simulink model "Drone_Model"  (R2021a)
settings: Solver=VariableStepAuto  StartTime=0.0  StopTime=10.0  MaxStep=1e-4  RelTol=1e-3
values from neighbouring files (symbols this model uses):
  g = 9.81    [Parameters.m]
  m = 0.8    [Parameters.m]
  Omega_sq_2_U = [b  b  b  b ... (first row only)    [Parameters.m]
  p1 = (Iyy-Izz)/Ixx    (= -0.808551372049)    [Parameters.m]
  p3 = l/Ixx    (= 19.1448627951)    [Parameters.m]
  p4 = (Izz-Ixx)/Iyy    (= 0.808551372049)    [Parameters.m]
  p6 = l/Iyy    (= 19.1448627951)    [Parameters.m]
  p7 = (Ixx-Iyy)/Izz    (= 0)    [Parameters.m]
  phi_0 = 0    [Parameters.m]
  phi_dot_0 = 0    [Parameters.m]
  psi_0 = 0    [Parameters.m]
  psi_dot_0 = 0    [Parameters.m]
  th_0 = 0    [Parameters.m]
  th_dot_0 = 0    [Parameters.m]
  U_Sq_max = U_max^2    (= 2467401.10027)    [Parameters.m]
  U_to_Omega_sq = inv(Omega_sq_2_U)    [Parameters.m]
  x_0 = 0.1    [Parameters.m]
  x_dot_0 = 0    [Parameters.m]
  y_0 = 0    [Parameters.m]
  y_dot_0 = 0    [Parameters.m]
  z_0 = 0    [Parameters.m]
  z_dot_0 = 0    [Parameters.m]
libraries: pid_lib x5
settings Model: Creator=jkord  LastModifiedBy=nikol
settings DebuggingCC: UnconnectedInputMsg=none  UnconnectedOutputMsg=none  UnconnectedLineMsg=none
settings ModelReferenceCC: EnableRefExpFcnMdlSchedulingChecks=off
settings RTWCC: Description=Generic Real-Time Target  GPUComputeCapability=5.0  DLArmComputeVersion=20.02.1

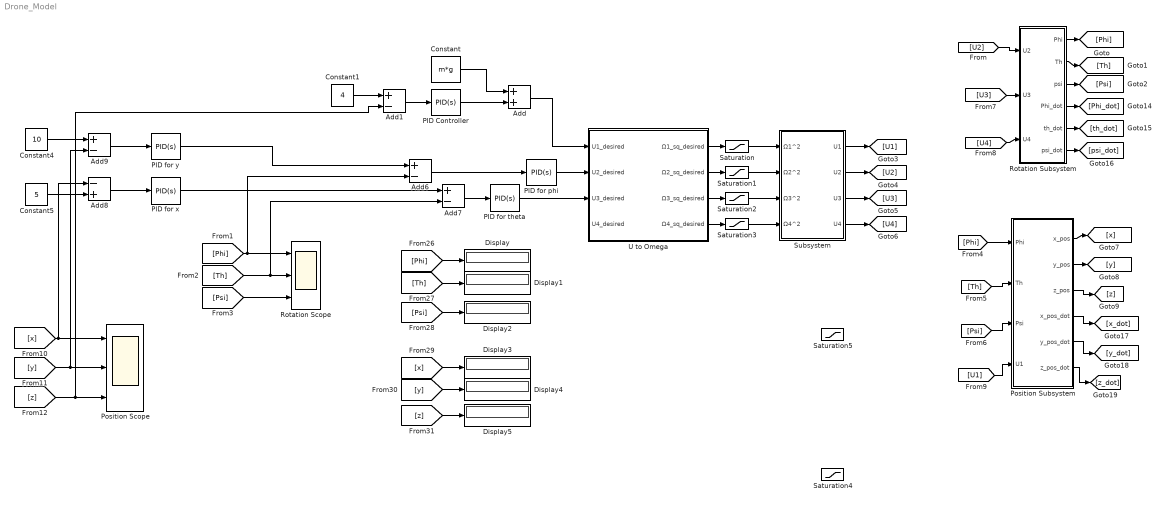
== system Drone_Model ==
  Add : Sum
  Add{1,6..7,9} (4 alike) : Sum  Inputs=+-
  Add8 : Sum  Inputs=-+
  Constant : Constant  Value=m*g
  Constant1 : Constant  Value=4
  Constant4 : Constant  Value=10
  Constant5 : Constant  Value=5
  Display{,1..5} (6 alike) : Display
  PID Controller : pid_lib/PID Controller  Controller=PID  Form=Parallel  TimeDomain=Continuous-time  UseExternalTs=off  SampleTime=-1  IntegratorMethod=Forward Euler  FilterMethod=Forward Euler  ControllerParametersSource=internal  P=0.81  I=0.875  D=0.9  UseFilter=on  N=100  TunerSelectOption=Frequency Response Based  InitialConditionSource=internal  InitialConditionForIntegrator=0  InitialConditionForFilter=0  DifferentiatorICPrevScaledInput=0  ExternalReset=none  TrackingMode=off  Kt=1  LimitOutput=off  SatLimitsSource=internal  UpperSaturationLimit=inf  LowerSaturationLimit=-inf  LinearizeAsGain=on  AntiWindupMode=none  Kb=1  POutMin=[]  POutMax=[]  IOutMin=[]  IOutMax=[]  DOutMin=[]  DOutMax=[]  NOutMin=[]  NOutMax=[]  SumOutMin=[]  SumOutMax=[]  SaturationOutMin=[]  SaturationOutMax=[]  PParamMin=[]  PParamMax=[]  IParamMin=[]  IParamMax=[]  DParamMin=[]  DParamMax=[]  NParamMin=[]  NParamMax=[]  KbParamMin=[]  KbParamMax=[]  KtParamMin=[]  KtParamMax=[]  KbOutMin=[]  KbOutMax=[]  KtOutMin=[]  KtOutMax=[]  IntegratorOutMin=[]  IntegratorOutMax=[]  FilterOutMin=[]  FilterOutMax=[]  SumI1OutMin=[]  SumI1OutMax=[]  SumI2OutMin=[]  SumI2OutMax=[]  SumI3OutMin=[]  SumI3OutMax=[]  SumI4OutMin=[]  SumI4OutMax=[]  SumDOutMin=[]  SumDOutMax=[]  DifferentiatorOutMin=[]  DifferentiatorOutMax=[]  FilterDiffOutCoefMin=[]  FilterDiffOutCoefMax=[]  ReciprocalOutMin=[]  ReciprocalOutMax=[]  SumDenOutMin=[]  SumDenOutMax=[]  SumNumOutMin=[]  SumNumOutMax=[]  DivideOutMin=[]  DivideOutMax=[]  UdiffTsProdOutMin=[]  UdiffTsProdOutMax=[]  NTsProdOutMin=[]  NTsProdOutMax=[]  UintegralTsProdOutMin=[]  UintegralTsProdOutMax=[]  UngainTsProdOutMin=[]  UngainTsProdOutMax=[]  IntegratorContinuousStateAttributes=''  IntegratorStateMustResolveToSignalObject=off  IntegratorRTWStateStorageClass=Auto  FilterContinuousStateAttributes=''  FilterStateMustResolveToSignalObject=off  FilterRTWStateStorageClass=Auto  ParallelPVariant=InternalParameters  IdealPVariant=Disabled  IVariant=InternalParameters  DVariant=InternalParameters  IntegratorVariant=Continuous  SatVariant=Disabled  AWVariant=Passthrough  PCopyVariant=Disabled  TRVariant=Disabled  FdbkBlocksVariant=Forward  IdealPFdbkVariant=Disabled  SatFdbkVariant=Disabled  DerivativeFilterVariant=ContFilter  NVariant=InternalParameters  NCopyVariant=Disabled  FilterICVariant=InternalICsFilter  IntegratorICVariant=InternalICs  ExternalResetVariant=Disabled  TRSumVariant=Passthrough  SumFdbkVariant=Disabled  SumVariant=Sum_PID  TsampFilterVariant=InternalTs  TsampNgainVariant=Passthrough  TsampIntegralVariant=Passthrough  ExternalSaturationOutDataTypeStr=Inherit: Same as second input
  PID for phi : pid_lib/PID Controller  Controller=PID  Form=Parallel  TimeDomain=Continuous-time  UseExternalTs=off  SampleTime=-1  IntegratorMethod=Forward Euler  FilterMethod=Forward Euler  ControllerParametersSource=internal  P=1  I=0.01  D=0.5  UseFilter=on  N=100  TunerSelectOption=Frequency Response Based  InitialConditionSource=internal  InitialConditionForIntegrator=0  InitialConditionForFilter=0  DifferentiatorICPrevScaledInput=0  ExternalReset=none  TrackingMode=off  Kt=1  LimitOutput=off  SatLimitsSource=internal  UpperSaturationLimit=inf  LowerSaturationLimit=-inf  LinearizeAsGain=on  AntiWindupMode=none  Kb=1  POutMin=[]  POutMax=[]  IOutMin=[]  IOutMax=[]  DOutMin=[]  DOutMax=[]  NOutMin=[]  NOutMax=[]  SumOutMin=[]  SumOutMax=[]  SaturationOutMin=[]  SaturationOutMax=[]  PParamMin=[]  PParamMax=[]  IParamMin=[]  IParamMax=[]  DParamMin=[]  DParamMax=[]  NParamMin=[]  NParamMax=[]  KbParamMin=[]  KbParamMax=[]  KtParamMin=[]  KtParamMax=[]  KbOutMin=[]  KbOutMax=[]  KtOutMin=[]  KtOutMax=[]  IntegratorOutMin=[]  IntegratorOutMax=[]  FilterOutMin=[]  FilterOutMax=[]  SumI1OutMin=[]  SumI1OutMax=[]  SumI2OutMin=[]  SumI2OutMax=[]  SumI3OutMin=[]  SumI3OutMax=[]  SumI4OutMin=[]  SumI4OutMax=[]  SumDOutMin=[]  SumDOutMax=[]  DifferentiatorOutMin=[]  DifferentiatorOutMax=[]  FilterDiffOutCoefMin=[]  FilterDiffOutCoefMax=[]  ReciprocalOutMin=[]  ReciprocalOutMax=[]  SumDenOutMin=[]  SumDenOutMax=[]  SumNumOutMin=[]  SumNumOutMax=[]  DivideOutMin=[]  DivideOutMax=[]  UdiffTsProdOutMin=[]  UdiffTsProdOutMax=[]  NTsProdOutMin=[]  NTsProdOutMax=[]  UintegralTsProdOutMin=[]  UintegralTsProdOutMax=[]  UngainTsProdOutMin=[]  UngainTsProdOutMax=[]  IntegratorContinuousStateAttributes=''  IntegratorStateMustResolveToSignalObject=off  IntegratorRTWStateStorageClass=Auto  FilterContinuousStateAttributes=''  FilterStateMustResolveToSignalObject=off  FilterRTWStateStorageClass=Auto  ParallelPVariant=InternalParameters  IdealPVariant=Disabled  IVariant=InternalParameters  DVariant=InternalParameters  IntegratorVariant=Continuous  SatVariant=Disabled  AWVariant=Passthrough  PCopyVariant=Disabled  TRVariant=Disabled  FdbkBlocksVariant=Forward  IdealPFdbkVariant=Disabled  SatFdbkVariant=Disabled  DerivativeFilterVariant=ContFilter  NVariant=InternalParameters  NCopyVariant=Disabled  FilterICVariant=InternalICsFilter  IntegratorICVariant=InternalICs  ExternalResetVariant=Disabled  TRSumVariant=Passthrough  SumFdbkVariant=Disabled  SumVariant=Sum_PID  TsampFilterVariant=InternalTs  TsampNgainVariant=Passthrough  TsampIntegralVariant=Passthrough  ExternalSaturationOutDataTypeStr=Inherit: Same as second input
  PID for theta : pid_lib/PID Controller  Controller=PID  Form=Parallel  TimeDomain=Continuous-time  UseExternalTs=off  SampleTime=-1  IntegratorMethod=Forward Euler  FilterMethod=Forward Euler  ControllerParametersSource=internal  P=0.75  I=0.16  D=0.12  UseFilter=on  N=100  TunerSelectOption=Frequency Response Based  InitialConditionSource=internal  InitialConditionForIntegrator=0  InitialConditionForFilter=0  DifferentiatorICPrevScaledInput=0  ExternalReset=none  TrackingMode=off  Kt=1  LimitOutput=off  SatLimitsSource=internal  UpperSaturationLimit=inf  LowerSaturationLimit=-inf  LinearizeAsGain=on  AntiWindupMode=none  Kb=1  POutMin=[]  POutMax=[]  IOutMin=[]  IOutMax=[]  DOutMin=[]  DOutMax=[]  NOutMin=[]  NOutMax=[]  SumOutMin=[]  SumOutMax=[]  SaturationOutMin=[]  SaturationOutMax=[]  PParamMin=[]  PParamMax=[]  IParamMin=[]  IParamMax=[]  DParamMin=[]  DParamMax=[]  NParamMin=[]  NParamMax=[]  KbParamMin=[]  KbParamMax=[]  KtParamMin=[]  KtParamMax=[]  KbOutMin=[]  KbOutMax=[]  KtOutMin=[]  KtOutMax=[]  IntegratorOutMin=[]  IntegratorOutMax=[]  FilterOutMin=[]  FilterOutMax=[]  SumI1OutMin=[]  SumI1OutMax=[]  SumI2OutMin=[]  SumI2OutMax=[]  SumI3OutMin=[]  SumI3OutMax=[]  SumI4OutMin=[]  SumI4OutMax=[]  SumDOutMin=[]  SumDOutMax=[]  DifferentiatorOutMin=[]  DifferentiatorOutMax=[]  FilterDiffOutCoefMin=[]  FilterDiffOutCoefMax=[]  ReciprocalOutMin=[]  ReciprocalOutMax=[]  SumDenOutMin=[]  SumDenOutMax=[]  SumNumOutMin=[]  SumNumOutMax=[]  DivideOutMin=[]  DivideOutMax=[]  UdiffTsProdOutMin=[]  UdiffTsProdOutMax=[]  NTsProdOutMin=[]  NTsProdOutMax=[]  UintegralTsProdOutMin=[]  UintegralTsProdOutMax=[]  UngainTsProdOutMin=[]  UngainTsProdOutMax=[]  IntegratorContinuousStateAttributes=''  IntegratorStateMustResolveToSignalObject=off  IntegratorRTWStateStorageClass=Auto  FilterContinuousStateAttributes=''  FilterStateMustResolveToSignalObject=off  FilterRTWStateStorageClass=Auto  ParallelPVariant=InternalParameters  IdealPVariant=Disabled  IVariant=InternalParameters  DVariant=InternalParameters  IntegratorVariant=Continuous  SatVariant=Disabled  AWVariant=Passthrough  PCopyVariant=Disabled  TRVariant=Disabled  FdbkBlocksVariant=Forward  IdealPFdbkVariant=Disabled  SatFdbkVariant=Disabled  DerivativeFilterVariant=ContFilter  NVariant=InternalParameters  NCopyVariant=Disabled  FilterICVariant=InternalICsFilter  IntegratorICVariant=InternalICs  ExternalResetVariant=Disabled  TRSumVariant=Passthrough  SumFdbkVariant=Disabled  SumVariant=Sum_PID  TsampFilterVariant=InternalTs  TsampNgainVariant=Passthrough  TsampIntegralVariant=Passthrough  ExternalSaturationOutDataTypeStr=Inherit: Same as second input
  PID for x : pid_lib/PID Controller  Controller=PID  Form=Parallel  TimeDomain=Continuous-time  UseExternalTs=off  SampleTime=-1  IntegratorMethod=Forward Euler  FilterMethod=Forward Euler  ControllerParametersSource=internal  P=1  I=.01  D=.25  UseFilter=on  N=100  TunerSelectOption=Frequency Response Based  InitialConditionSource=internal  InitialConditionForIntegrator=0  InitialConditionForFilter=0  DifferentiatorICPrevScaledInput=0  ExternalReset=none  TrackingMode=off  Kt=1  LimitOutput=off  SatLimitsSource=internal  UpperSaturationLimit=inf  LowerSaturationLimit=-inf  LinearizeAsGain=on  AntiWindupMode=none  Kb=1  POutMin=[]  POutMax=[]  IOutMin=[]  IOutMax=[]  DOutMin=[]  DOutMax=[]  NOutMin=[]  NOutMax=[]  SumOutMin=[]  SumOutMax=[]  SaturationOutMin=[]  SaturationOutMax=[]  PParamMin=[]  PParamMax=[]  IParamMin=[]  IParamMax=[]  DParamMin=[]  DParamMax=[]  NParamMin=[]  NParamMax=[]  KbParamMin=[]  KbParamMax=[]  KtParamMin=[]  KtParamMax=[]  KbOutMin=[]  KbOutMax=[]  KtOutMin=[]  KtOutMax=[]  IntegratorOutMin=[]  IntegratorOutMax=[]  FilterOutMin=[]  FilterOutMax=[]  SumI1OutMin=[]  SumI1OutMax=[]  SumI2OutMin=[]  SumI2OutMax=[]  SumI3OutMin=[]  SumI3OutMax=[]  SumI4OutMin=[]  SumI4OutMax=[]  SumDOutMin=[]  SumDOutMax=[]  DifferentiatorOutMin=[]  DifferentiatorOutMax=[]  FilterDiffOutCoefMin=[]  FilterDiffOutCoefMax=[]  ReciprocalOutMin=[]  ReciprocalOutMax=[]  SumDenOutMin=[]  SumDenOutMax=[]  SumNumOutMin=[]  SumNumOutMax=[]  DivideOutMin=[]  DivideOutMax=[]  UdiffTsProdOutMin=[]  UdiffTsProdOutMax=[]  NTsProdOutMin=[]  NTsProdOutMax=[]  UintegralTsProdOutMin=[]  UintegralTsProdOutMax=[]  UngainTsProdOutMin=[]  UngainTsProdOutMax=[]  IntegratorContinuousStateAttributes=''  IntegratorStateMustResolveToSignalObject=off  IntegratorRTWStateStorageClass=Auto  FilterContinuousStateAttributes=''  FilterStateMustResolveToSignalObject=off  FilterRTWStateStorageClass=Auto  ParallelPVariant=InternalParameters  IdealPVariant=Disabled  IVariant=InternalParameters  DVariant=InternalParameters  IntegratorVariant=Continuous  SatVariant=Disabled  AWVariant=Passthrough  PCopyVariant=Disabled  TRVariant=Disabled  FdbkBlocksVariant=Forward  IdealPFdbkVariant=Disabled  SatFdbkVariant=Disabled  DerivativeFilterVariant=ContFilter  NVariant=InternalParameters  NCopyVariant=Disabled  FilterICVariant=InternalICsFilter  IntegratorICVariant=InternalICs  ExternalResetVariant=Disabled  TRSumVariant=Passthrough  SumFdbkVariant=Disabled  SumVariant=Sum_PID  TsampFilterVariant=InternalTs  TsampNgainVariant=Passthrough  TsampIntegralVariant=Passthrough  ExternalSaturationOutDataTypeStr=Inherit: Same as second input
  PID for y : pid_lib/PID Controller  Controller=PID  Form=Parallel  TimeDomain=Continuous-time  UseExternalTs=off  SampleTime=-1  IntegratorMethod=Forward Euler  FilterMethod=Forward Euler  ControllerParametersSource=internal  P=0.6  I=0  D=0.3  UseFilter=on  N=100  TunerSelectOption=Frequency Response Based  InitialConditionSource=internal  InitialConditionForIntegrator=0  InitialConditionForFilter=0  DifferentiatorICPrevScaledInput=0  ExternalReset=none  TrackingMode=off  Kt=1  LimitOutput=off  SatLimitsSource=internal  UpperSaturationLimit=inf  LowerSaturationLimit=-inf  LinearizeAsGain=on  AntiWindupMode=none  Kb=1  POutMin=[]  POutMax=[]  IOutMin=[]  IOutMax=[]  DOutMin=[]  DOutMax=[]  NOutMin=[]  NOutMax=[]  SumOutMin=[]  SumOutMax=[]  SaturationOutMin=[]  SaturationOutMax=[]  PParamMin=[]  PParamMax=[]  IParamMin=[]  IParamMax=[]  DParamMin=[]  DParamMax=[]  NParamMin=[]  NParamMax=[]  KbParamMin=[]  KbParamMax=[]  KtParamMin=[]  KtParamMax=[]  KbOutMin=[]  KbOutMax=[]  KtOutMin=[]  KtOutMax=[]  IntegratorOutMin=[]  IntegratorOutMax=[]  FilterOutMin=[]  FilterOutMax=[]  SumI1OutMin=[]  SumI1OutMax=[]  SumI2OutMin=[]  SumI2OutMax=[]  SumI3OutMin=[]  SumI3OutMax=[]  SumI4OutMin=[]  SumI4OutMax=[]  SumDOutMin=[]  SumDOutMax=[]  DifferentiatorOutMin=[]  DifferentiatorOutMax=[]  FilterDiffOutCoefMin=[]  FilterDiffOutCoefMax=[]  ReciprocalOutMin=[]  ReciprocalOutMax=[]  SumDenOutMin=[]  SumDenOutMax=[]  SumNumOutMin=[]  SumNumOutMax=[]  DivideOutMin=[]  DivideOutMax=[]  UdiffTsProdOutMin=[]  UdiffTsProdOutMax=[]  NTsProdOutMin=[]  NTsProdOutMax=[]  UintegralTsProdOutMin=[]  UintegralTsProdOutMax=[]  UngainTsProdOutMin=[]  UngainTsProdOutMax=[]  IntegratorContinuousStateAttributes=''  IntegratorStateMustResolveToSignalObject=off  IntegratorRTWStateStorageClass=Auto  FilterContinuousStateAttributes=''  FilterStateMustResolveToSignalObject=off  FilterRTWStateStorageClass=Auto  ParallelPVariant=InternalParameters  IdealPVariant=Disabled  IVariant=InternalParameters  DVariant=InternalParameters  IntegratorVariant=Continuous  SatVariant=Disabled  AWVariant=Passthrough  PCopyVariant=Disabled  TRVariant=Disabled  FdbkBlocksVariant=Forward  IdealPFdbkVariant=Disabled  SatFdbkVariant=Disabled  DerivativeFilterVariant=ContFilter  NVariant=InternalParameters  NCopyVariant=Disabled  FilterICVariant=InternalICsFilter  IntegratorICVariant=InternalICs  ExternalResetVariant=Disabled  TRSumVariant=Passthrough  SumFdbkVariant=Disabled  SumVariant=Sum_PID  TsampFilterVariant=InternalTs  TsampNgainVariant=Passthrough  TsampIntegralVariant=Passthrough  ExternalSaturationOutDataTypeStr=Inherit: Same as second input
  Position Subsystem : Subsystem
  Position Scope : Scope  NumInputPorts=3
  Rotation Subsystem : Subsystem
  Rotation Scope : Scope  NumInputPorts=3
  Saturation{,1..5} (6 alike) : Saturate  UpperLimit=U_Sq_max  LowerLimit=0
  Subsystem : Subsystem
  U to Omega : Subsystem
  wires:
  [Th] -> Position Subsystem/2(Th)
  [U3] -> Rotation Subsystem/2(U3)
  Rotation Subsystem/3(psi) -> [Psi]
  [U4] -> Rotation Subsystem/3(U4)
  Rotation Subsystem/1(Phi) -> [Phi]
  Rotation Subsystem/6(psi_dot) -> [psi_dot]
  Rotation Subsystem/2(Th) -> [Th]
  Position Subsystem/6(z_pos_dot) -> [z_dot]
  [Phi] -> Position Subsystem/1(Phi)
  Rotation Subsystem/4(Phi_dot) -> [Phi_dot]
  Rotation Subsystem/5(th_dot) -> [th_dot]
  Position Subsystem/4(x_pos_dot) -> [x_dot]
  [Psi] -> Position Subsystem/3(Psi)
  Position Subsystem/5(y_pos_dot) -> [y_dot]
  Position Subsystem/1(x_pos) -> [x]
  [U1] -> Position Subsystem/4(U1)
  Position Subsystem/3(z_pos) -> [z]
  Position Subsystem/2(y_pos) -> [y]
  [U2] -> Rotation Subsystem/1(U2)
  U to Omega/1(Ω1_sq_desired) -> Saturation/1
  Saturation3/1 -> Subsystem/4(Ω4^2)
  U to Omega/3(Ω3_sq_desired) -> Saturation2/1
  U to Omega/2(Ω2_sq_desired) -> Saturation1/1
  Saturation2/1 -> Subsystem/3(Ω3^2)
  Saturation1/1 -> Subsystem/2(Ω2^2)
  U to Omega/4(Ω4_sq_desired) -> Saturation3/1
  Subsystem/4(U4) -> [U4]
  Saturation/1 -> Subsystem/1(Ω1^2)
  Subsystem/2(U2) -> [U2]
  Subsystem/3(U3) -> [U3]
  Subsystem/1(U1) -> [U1]
  [Psi] -> Rotation Scope/3
  [z] -> Display5/1
  [Psi] -> Display2/1
  [Th] -> Display1/1
  [Phi] -> Display/1
  [x] -> Display3/1
  [y] -> Display4/1
  PID Controller/1 -> Add/2
  Constant/1 -> Add/1
  Add1/1 -> PID Controller/1
  Constant1/1 -> Add1/1
  [z] -> Add1/2, Position Scope/3
  Add/1 -> U to Omega/1(U1_desired)
  PID for theta/1 -> U to Omega/3(U3_desired)
  PID for phi/1 -> U to Omega/2(U2_desired)
  PID for y/1 -> Add6/1
  Add6/1 -> PID for phi/1
  [Phi] -> Rotation Scope/1, Add6/2
  Add7/1 -> PID for theta/1
  PID for x/1 -> Add7/1
  [Th] -> Add7/2, Rotation Scope/2
  [x] -> Add8/1, Position Scope/1
  [y] -> Add9/2, Position Scope/2
  Constant5/1 -> Add8/2
  Constant4/1 -> Add9/1
  Add9/1 -> PID for y/1
  Add8/1 -> PID for x/1

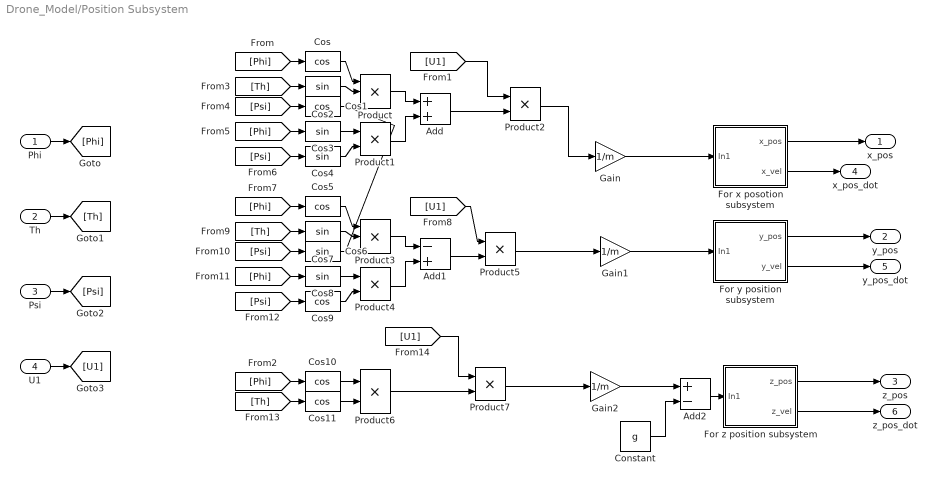
== system Drone_Model/Position Subsystem ==
  Phi : Inport
  Th : Inport  Port=2
  Psi : Inport  Port=3
  U1 : Inport  Port=4
  Add : Sum
  Add1 : Sum  Inputs=-+
  Add2 : Sum  Inputs=+-
  Constant : Constant  Value=g
  Cos{,1,5,9..11} (6 alike) : Trigonometry  Operator=cos
  Cos{2..4,6..8} (6 alike) : Trigonometry
  For x posotion subsystem : Subsystem
  For y position subsystem : Subsystem
  For z position subsystem : Subsystem
  Gain : Gain  Gain=1/m
  Gain1 : Gain  Gain=1/m
  Gain2 : Gain  Gain=1/m
  Product : Product  Inputs=3
  Product{1..2,4..7} (6 alike) : Product
  Product3 : Product  Inputs=3
  x_pos : Outport
  y_pos : Outport  Port=2
  z_pos : Outport  Port=3
  x_pos_dot : Outport  Port=4
  y_pos_dot : Outport  Port=5
  z_pos_dot : Outport  Port=6
  wires:
  For z position subsystem/1(z_pos) -> z_pos/1
  For z position subsystem/2(z_vel) -> z_pos_dot/1
  For x posotion subsystem/1(x_pos) -> x_pos/1
  For y position subsystem/1(y_pos) -> y_pos/1
  For y position subsystem/2(y_vel) -> y_pos_dot/1
  Phi/1 -> [Phi]
  Th/1 -> [Th]
  Psi/1 -> [Psi]
  [Phi] -> Cos/1
  [Psi] -> Cos1/1
  [Th] -> Cos2/1
  Cos2/1 -> Product/2
  Cos/1 -> Product/1
  Cos1/1 -> ?
  Product/1 -> Add/1
  [Phi] -> Cos3/1
  [Psi] -> Cos4/1
  Cos3/1 -> Product1/1
  Cos4/1 -> Product1/2
  Product1/1 -> Add/2
  U1/1 -> [U1]
  [U1] -> Product2/1
  Add/1 -> Product2/2
  Product2/1 -> Gain/1
  Gain/1 -> For x posotion subsystem/1(In1)
  [Phi] -> Cos5/1
  [Psi] -> Cos6/1
  [Phi] -> Cos8/1
  Cos6/1 -> ?
  Add1/1 -> Product5/2
  Gain1/1 -> For y position subsystem/1(In1)
  [Psi] -> Cos9/1
  Product4/1 -> Add1/2
  [U1] -> Product5/1
  Product3/1 -> Add1/1
  Cos5/1 -> Product3/1
  Cos7/1 -> Product3/2
  Cos9/1 -> Product4/2
  Cos8/1 -> Product4/1
  [Th] -> Cos7/1
  Product5/1 -> Gain1/1
  Add2/1 -> For z position subsystem/1(In1)
  [Phi] -> Cos10/1
  Cos10/1 -> Product6/1
  Cos11/1 -> Product6/2
  [Th] -> Cos11/1
  [U1] -> Product7/1
  Product6/1 -> Product7/2
  Gain2/1 -> Add2/1
  Product7/1 -> Gain2/1
  Constant/1 -> Add2/2
  For x posotion subsystem/2(x_vel) -> x_pos_dot/1

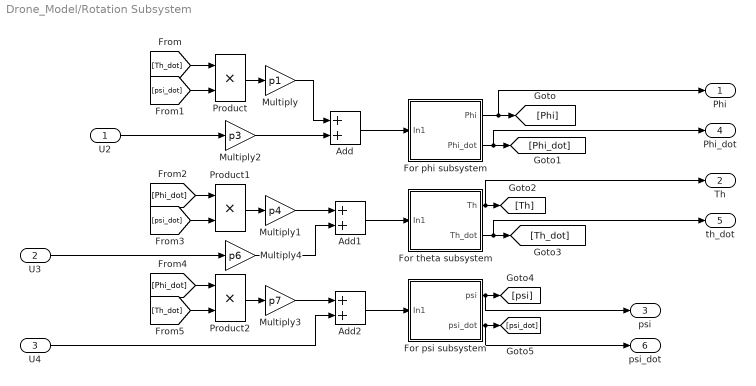
== system Drone_Model/Rotation Subsystem ==
  U2 : Inport
  U3 : Inport  Port=2
  U4 : Inport  Port=3
  Add : Sum
  Add1 : Sum
  Add2 : Sum
  For phi subsystem : Subsystem
  For psi subsystem : Subsystem
  For theta subsystem : Subsystem
  Multiply : Gain  Gain=p1
  Multiply1 : Gain  Gain=p4
  Multiply2 : Gain  Gain=p3
  Multiply3 : Gain  Gain=p7
  Multiply4 : Gain  Gain=p6
  Product : Product
  Product1 : Product
  Product2 : Product
  Phi : Outport
  Th : Outport  Port=2
  psi : Outport  Port=3
  Phi_dot : Outport  Port=4
  th_dot : Outport  Port=5
  psi_dot : Outport  Port=6
  wires:
  For psi subsystem/1(psi) -> psi/1, [psi]
  [psi_dot] -> Product1/2
  For psi subsystem/2(psi_dot) -> psi_dot/1, [psi_dot]
  Multiply2/1 -> Add/2
  For phi subsystem/2(Phi_dot) -> Phi_dot/1, [Phi_dot]
  For phi subsystem/1(Phi) -> Phi/1, [Phi]
  Product/1 -> Multiply/1
  For theta subsystem/1(Th) -> Th/1, [Th]
  Product1/1 -> Multiply1/1
  [Phi_dot] -> Product1/1
  Multiply/1 -> Add/1
  Add/1 -> For phi subsystem/1(In1)
  [Th_dot] -> Product2/2
  Add2/1 -> For psi subsystem/1(In1)
  Multiply1/1 -> Add1/1
  [psi_dot] -> Product/2
  For theta subsystem/2(Th_dot) -> th_dot/1, [Th_dot]
  Multiply3/1 -> Add2/1
  [Th_dot] -> Product/1
  Add1/1 -> For theta subsystem/1(In1)
  [Phi_dot] -> Product2/1
  Product2/1 -> Multiply3/1
  U3/1 -> Multiply4/1
  U2/1 -> Multiply2/1
  U4/1 -> Add2/2
  Multiply4/1 -> Add1/2

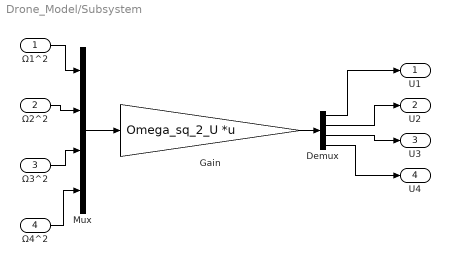
== system Drone_Model/Subsystem ==
  Ω1^2 : Inport
  Ω2^2 : Inport  Port=2
  Ω3^2 : Inport  Port=3
  Ω4^2 : Inport  Port=4
  Demux : Demux
  Gain : Gain  Gain=Omega_sq_2_U  Multiplication=Matrix(K*u)
  Mux : Mux
  U1 : Outport
  U2 : Outport  Port=2
  U3 : Outport  Port=3
  U4 : Outport  Port=4
  wires:
  Ω2^2/1 -> Mux/2
  Ω3^2/1 -> Mux/3
  Ω1^2/1 -> Mux/1
  Ω4^2/1 -> Mux/4
  Mux/1 -> Gain/1
  Gain/1 -> Demux/1
  Demux/1 -> U1/1
  Demux/2 -> U2/1
  Demux/3 -> U3/1
  Demux/4 -> U4/1

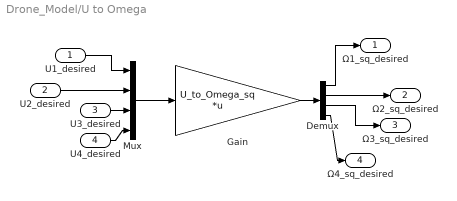
== system Drone_Model/U to Omega ==
  U1_desired : Inport
  U2_desired : Inport  Port=2
  U3_desired : Inport  Port=3
  U4_desired : Inport  Port=4
  Demux : Demux
  Gain : Gain  Gain=U_to_Omega_sq  Multiplication=Matrix(K*u)
  Mux : Mux
  Ω1_sq_desired : Outport
  Ω2_sq_desired : Outport  Port=2
  Ω3_sq_desired : Outport  Port=3
  Ω4_sq_desired : Outport  Port=4
  wires:
  U4_desired/1 -> Mux/4
  U1_desired/1 -> Mux/1
  Demux/3 -> Ω3_sq_desired/1
  Mux/1 -> Gain/1
  Demux/2 -> Ω2_sq_desired/1
  U2_desired/1 -> Mux/2
  Demux/4 -> Ω4_sq_desired/1
  U3_desired/1 -> Mux/3
  Demux/1 -> Ω1_sq_desired/1
  Gain/1 -> Demux/1

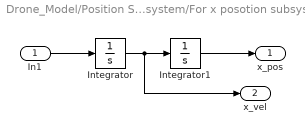
== system Drone_Model/Position Subsystem/For x posotion subsystem ==
  In1 : Inport
  Integrator : Integrator  InitialCondition=x_dot_0
  Integrator1 : Integrator  InitialCondition=x_0
  x_pos : Outport
  x_vel : Outport  Port=2
  wires:
  Integrator/1 -> x_vel/1, Integrator1/1
  In1/1 -> Integrator/1
  Integrator1/1 -> x_pos/1

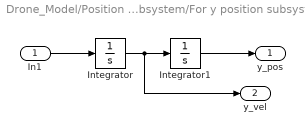
== system Drone_Model/Position Subsystem/For y position subsystem ==
  In1 : Inport
  Integrator : Integrator  InitialCondition=y_dot_0
  Integrator1 : Integrator  InitialCondition=y_0
  y_pos : Outport
  y_vel : Outport  Port=2
  wires:
  Integrator1/1 -> y_pos/1
  In1/1 -> Integrator/1
  Integrator/1 -> Integrator1/1, y_vel/1

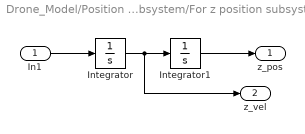
== system Drone_Model/Position Subsystem/For z position subsystem ==
  In1 : Inport
  Integrator : Integrator  InitialCondition=z_dot_0
  Integrator1 : Integrator  InitialCondition=z_0
  z_pos : Outport
  z_vel : Outport  Port=2
  wires:
  Integrator/1 -> z_vel/1, Integrator1/1
  In1/1 -> Integrator/1
  Integrator1/1 -> z_pos/1

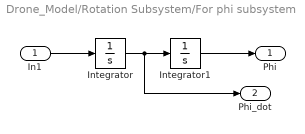
== system Drone_Model/Rotation Subsystem/For phi subsystem ==
  In1 : Inport
  Integrator : Integrator  InitialCondition=phi_dot_0
  Integrator1 : Integrator  InitialCondition=phi_0
  Phi : Outport
  Phi_dot : Outport  Port=2
  wires:
  Integrator/1 -> Phi_dot/1, Integrator1/1
  In1/1 -> Integrator/1
  Integrator1/1 -> Phi/1

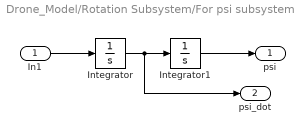
== system Drone_Model/Rotation Subsystem/For psi subsystem ==
  In1 : Inport
  Integrator : Integrator  InitialCondition=psi_dot_0
  Integrator1 : Integrator  InitialCondition=psi_0
  psi : Outport
  psi_dot : Outport  Port=2
  wires:
  Integrator/1 -> psi_dot/1, Integrator1/1
  In1/1 -> Integrator/1
  Integrator1/1 -> psi/1

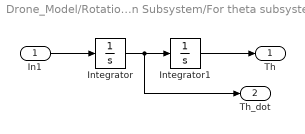
== system Drone_Model/Rotation Subsystem/For theta subsystem ==
  In1 : Inport
  Integrator : Integrator  InitialCondition=th_dot_0
  Integrator1 : Integrator  InitialCondition=th_0
  Th : Outport
  Th_dot : Outport  Port=2
  wires:
  Integrator1/1 -> Th/1
  In1/1 -> Integrator/1
  Integrator/1 -> Integrator1/1, Th_dot/1
